simulink model "Brown_Homework7_Trim_Helper"  (R2025b)
settings: Solver=ode45  StartTime=0.0  StopTime=1  RelTol=1e-3
values from neighbouring files (symbols this model uses):
  trim_cruise_tilt_deg = cruiseTiltDeg    (= 90)    [HOMEWORK7_trim_linmod_live_source.m]
  trim_target_bank_deg = banks(k)    [HOMEWORK7_trim_linmod_live_source.m]
  trim_target_speed_mps = speeds(k)    [HOMEWORK7_trim_linmod_live_source.m]
undefined symbols (not defined in the file or in its folder): trim_residual_component
settings Model: Creator=zbrown  LastModifiedBy=zbrown
settings DataIOCC: SaveOutput=off  SaveTime=off

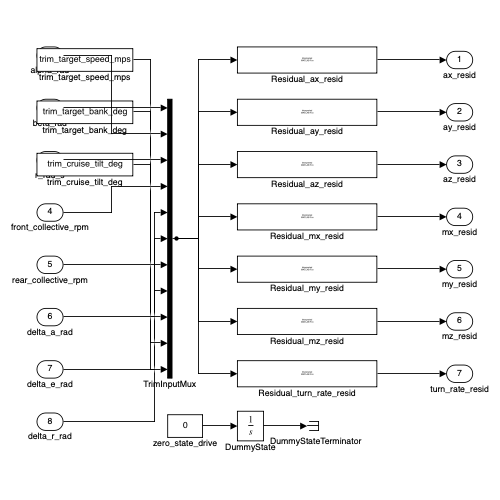
[thumbnail: Simulink's stored preview of the top-level diagram]
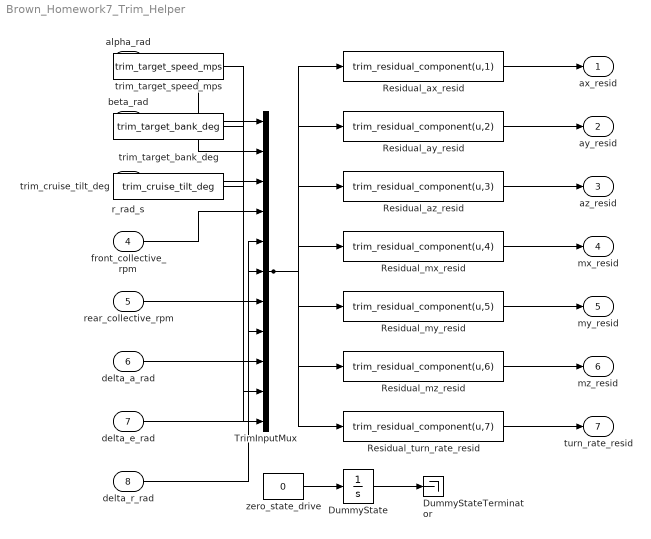
== system Brown_Homework7_Trim_Helper ==
  alpha_rad : Inport
  beta_rad : Inport  Port=2
  r_rad_s : Inport  Port=3
  front_collective_rpm : Inport  Port=4
  rear_collective_rpm : Inport  Port=5
  delta_a_rad : Inport  Port=6
  delta_e_rad : Inport  Port=7
  delta_r_rad : Inport  Port=8
  DummyState : Integrator
  DummyStateTerminator : Terminator
  Residual_ax_resid : MATLABFcn  MATLABFcn=trim_residual_component(u,1)
  Residual_ay_resid : MATLABFcn  MATLABFcn=trim_residual_component(u,2)
  Residual_az_resid : MATLABFcn  MATLABFcn=trim_residual_component(u,3)
  Residual_mx_resid : MATLABFcn  MATLABFcn=trim_residual_component(u,4)
  Residual_my_resid : MATLABFcn  MATLABFcn=trim_residual_component(u,5)
  Residual_mz_resid : MATLABFcn  MATLABFcn=trim_residual_component(u,6)
  Residual_turn_rate_resid : MATLABFcn  MATLABFcn=trim_residual_component(u,7)
  TrimInputMux : Mux  Inputs=11
  trim_cruise_tilt_deg : Constant  Value=trim_cruise_tilt_deg
  trim_target_bank_deg : Constant  Value=trim_target_bank_deg
  trim_target_speed_mps : Constant  Value=trim_target_speed_mps
  zero_state_drive : Constant  Value=0
  ax_resid : Outport
  ay_resid : Outport  Port=2
  az_resid : Outport  Port=3
  mx_resid : Outport  Port=4
  my_resid : Outport  Port=5
  mz_resid : Outport  Port=6
  turn_rate_resid : Outport  Port=7
  wires:
  alpha_rad/1 -> TrimInputMux/1
  beta_rad/1 -> TrimInputMux/2
  r_rad_s/1 -> TrimInputMux/3
  front_collective_rpm/1 -> TrimInputMux/4
  rear_collective_rpm/1 -> TrimInputMux/5
  delta_a_rad/1 -> TrimInputMux/6
  delta_e_rad/1 -> TrimInputMux/7
  delta_r_rad/1 -> TrimInputMux/8
  trim_target_speed_mps/1 -> TrimInputMux/9
  trim_target_bank_deg/1 -> TrimInputMux/10
  trim_cruise_tilt_deg/1 -> TrimInputMux/11
  TrimInputMux/1 -> Residual_ax_resid/1, Residual_ay_resid/1, Residual_az_resid/1, Residual_mx_resid/1, Residual_my_resid/1, Residual_mz_resid/1, Residual_turn_rate_resid/1
  Residual_ax_resid/1 -> ax_resid/1
  Residual_ay_resid/1 -> ay_resid/1
  Residual_az_resid/1 -> az_resid/1
  Residual_mx_resid/1 -> mx_resid/1
  Residual_my_resid/1 -> my_resid/1
  Residual_mz_resid/1 -> mz_resid/1
  Residual_turn_rate_resid/1 -> turn_rate_resid/1
  zero_state_drive/1 -> DummyState/1
  DummyState/1 -> DummyStateTerminator/1
